simulink model "LWR4"  (R2014a)
settings: Solver=ode4  StartTime=0  StopTime=30  FixedStep=0.05  MaxStep=0.010  RelTol=1e-3
InitFcn:
  | clear all
  | clc
  | 
  | global clientID
  | global vrep
  | global vecJoints nJoints
  | 
  | Rob_KUKA_LWR4plus_Jacobian
  | 
  | load_path
  | KP= diag([1,1,1,1,1,1,1])
  | KI= diag([1,1,1,1,1,1,1])
  | 
  | addpath('C:\Program Files (x86)\V-REP3\V-REP_PRO_EDU\programming\remoteApiBindings\lib\lib\64Bit')
  | 
  | 
  | disp('Program started');
  | vrep=remApi('remoteApi'); % using the prototype file (remoteApiProto.m)
  | vrep.simxFinish(-1); % just in case, close all opened connections
  | clientID=vrep.simxStart('127.0.0.1',19997,true,true,5000,5);
  | 
  | vrep.simxStartSimulation(clientID,vrep.simx_opmode_oneshot_wait);
  | vrep.simxSynchronous(clientID,true)
  | 
  | if (clientID<=-1)
  |     disp('stop simulation')
  |     vrep.delete();
  |     set_param(gcs, 'SimulationCommand', 'stop')
  | end
  | 
  | % Root of the joint in Vrep
  | rootJoints     = 'LBR4p_joint';
  | 
  | % Number of joints
  | nJoints        = 7;
  | 
  | % Handles of the joints
  | vecJoints      = zeros(nJoints,1);
  | 
  | for i=1:nJoints
  |                 [res,obj]=vrep.simxGetObjectHandle(clientID,strcat(rootJoints,int2str(i)),vrep.simx_opmode_oneshot_wait);
  |                 if res==vrep.simx_return_ok
  |                     vecJoints(i) = obj;
  |                    [res,pos] = vrep.simxGetJointPosition(clientID,vecJoints(i),vrep.simx_opmode_streaming);
  |                 else
  |                     vecJoints(i) = -1;
  |                     disp(strcat('joint nr ', int2str(i), ' named ', rootJoints, int2str(i) , ' not avalaible!'));
  |                 end
  | end
StopFcn:
  | global clientID
  | 
  | vrep.simxStopSimulation(clientID,vrep.simx_opmode_oneshot_wait);
settings Model: Creator=Massimo  LastModifiedBy=Admin
settings DebuggingCC: UnderspecifiedInitializationDetection=Classic  SolverPrmCheckMsg=none  StateNameClashWarn=warning

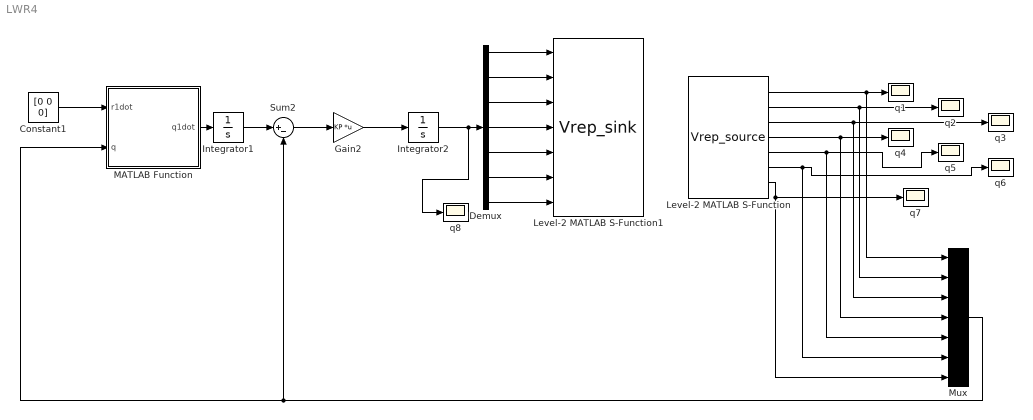
== system LWR4 ==
  Constant1 : Constant  Value=[0 0 0]
  Demux : Demux  Outputs=7
  Gain2 : Gain  Gain=KP  Multiplication=Matrix(K*u)
  Integrator1 : Integrator
  Integrator2 : Integrator
  Level-2 MATLAB S-Function : M-S-Function  FunctionName=Vrep_source
  Level-2 MATLAB S-Function1 : M-S-Function  FunctionName=Vrep_sink
  MATLAB Function : MATLAB Function  TreatAsAtomicUnit=on
  Mux : Mux  Inputs=7
  Sum2 : Sum  Inputs=|+-
  q{1..8} (8 alike) : Scope
      q1 settings: YMin=2.965  YMax=2.9695
      q3 settings: SaveName=ScopeData2
      q4 settings: SaveName=ScopeData3
      q5 settings: SaveName=ScopeData4
      q6 settings: SaveName=ScopeData5
      q7 settings: SaveName=ScopeData6
      q8 settings: TimeRange=12  YMin=-2.9745  YMax=-2.967  SaveName=ScopeData7
  wires:
  Level-2 MATLAB S-Function/1 -> Mux/1, q1/1
  Level-2 MATLAB S-Function/2 -> Mux/2, q2/1
  Level-2 MATLAB S-Function/3 -> Mux/3, q3/1
  Level-2 MATLAB S-Function/4 -> Mux/4, q4/1
  Level-2 MATLAB S-Function/5 -> Mux/5, q5/1
  Level-2 MATLAB S-Function/6 -> Mux/6, q6/1
  Level-2 MATLAB S-Function/7 -> Mux/7, q7/1
  Demux/4 -> Level-2 MATLAB S-Function1/4
  Demux/5 -> Level-2 MATLAB S-Function1/5
  Demux/3 -> Level-2 MATLAB S-Function1/3
  Demux/2 -> Level-2 MATLAB S-Function1/2
  Demux/1 -> Level-2 MATLAB S-Function1/1
  Demux/6 -> Level-2 MATLAB S-Function1/6
  Demux/7 -> Level-2 MATLAB S-Function1/7
  Gain2/1 -> Integrator2/1
  Mux/1 -> Sum2/2, MATLAB Function/2(q)
  MATLAB Function/1(q1dot) -> Integrator1/1
  Integrator1/1 -> Sum2/1
  Sum2/1 -> Gain2/1
  Constant1/1 -> MATLAB Function/1(r1dot)
  Integrator2/1 -> q8/1, Demux/1

== matlab function LWR4/MATLAB Function ==
  data: r1dot input; q input; q1dot output size=7
function q1dot = J1pinv(r1dot,q)
q1=q(1);
q2=q(2);
q3=q(3);
q4=q(4);
q5=q(5);
q6=q(6);
q7=q(7);
J=[ 0, -79/100, 0, 39/100, 0,  0, 0
 0,       0, 0,      0, 0,  0, 0
 0,       0, 0,      0, 0,  0, 0]
Jpinv=pinv(J)
q1dot=Jpinv*r1dot
